simulink model "ILC_Intro_Saturate"  (R2017a)
settings: Solver=VariableStepAuto  StartTime=0.0  StopTime=10.0  RelTol=1e-3
undefined symbols (not defined in the file or in its folder): K, umax
libraries: cstblocks x1
settings Model: Creator=capn  LastModifiedBy=capn

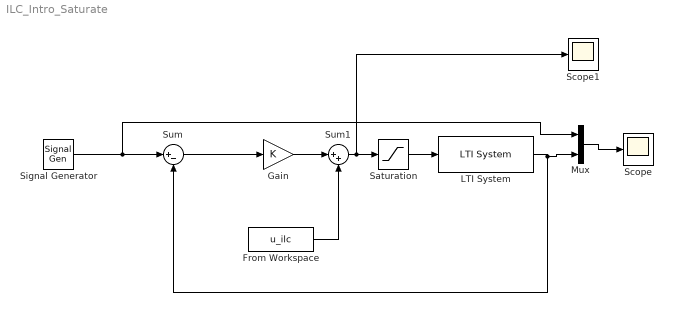
== system ILC_Intro_Saturate ==
  From Workspace : FromWorkspace  VariableName=u_ilc  SampleTime=0
  Gain : Gain  Gain=K
  LTI System : cstblocks/LTI System  sys=Pd  IC=[]
  Mux : Mux  Inputs=2
  Saturation : Saturate  UpperLimit=umax  LowerLimit=-umax
  Scope : Scope
  Scope1 : Scope
  Signal Generator : SignalGenerator  WaveForm=square  Units=rad/sec
  Sum : Sum  Inputs=|+-
  Sum1 : Sum  Inputs=|++
  wires:
  Sum/1 -> Gain/1
  Gain/1 -> Sum1/1
  Sum1/1 -> Saturation/1, Scope1/1
  Signal Generator/1 -> Mux/1, Sum/1
  From Workspace/1 -> Sum1/2
  LTI System/1 -> Mux/2, Sum/2
  Mux/1 -> Scope/1
  Saturation/1 -> LTI System/1
